simulink model "system_level_worst_case"  (R2025a)
settings: Solver=VariableStepAuto  StartTime=0.0  StopTime=350  RelTol=1e-3
libraries: simulink x5
settings Model: PacingRate=10  Creator=lynnyu  LastModifiedBy=lynnyu

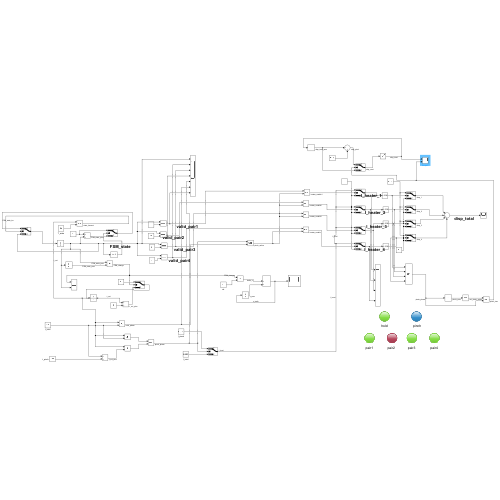
[thumbnail: Simulink's stored preview of the top-level diagram]
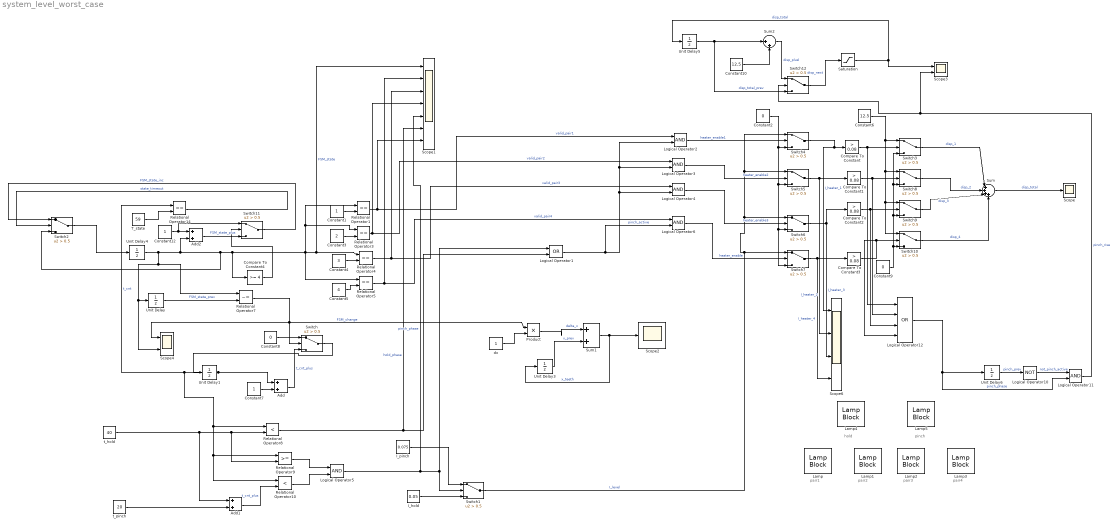
== system system_level_worst_case ==
  note: pair1
  note: pair2
  note: pair3
  note: pair4
  note: hold
  note: pinch
  Add : Sum
  Add1 : Sum
  Add2 : Sum
  Compare To Constant{,1..3} (4 alike) : simulink/Logic and Bit Operations/Compare To Constant  relop=>  const=0.08  OutDataTypeStr=boolean
  Compare To Constant4 : simulink/Logic and Bit Operations/Compare To Constant  relop=>=  const=4  OutDataTypeStr=boolean
  Constant1 : Constant
  Constant10 : Constant  Value=12.5
  Constant12 : Constant
  Constant2 : Constant  Value=0
  Constant3 : Constant  Value=2
  Constant4 : Constant  Value=3
  Constant5 : Constant  Value=4
  Constant6 : Constant  Value=12.5
  Constant7 : Constant
  Constant8 : Constant  Value=0
  Constant9 : Constant  Value=0
  I_hold : Constant  Value=0.05
  I_pinch : Constant  Value=0.075
  Lamp{,1..5} (6 alike) : LampBlock  LabelPosition=Hide  DefaultColor=[192.0, 192.0, 192.0]
  Logical Operator1 : Logic  Operator=OR  AllPortsSameDT=off  OutDataTypeStr=boolean
  Logical Operator10 : Logic  Operator=NOT  AllPortsSameDT=off  OutDataTypeStr=boolean
  Logical Operator{2..6,11} (6 alike) : Logic  AllPortsSameDT=off  OutDataTypeStr=boolean
  Logical Operator12 : Logic  Operator=OR  Inputs=4  AllPortsSameDT=off  OutDataTypeStr=boolean
  Product : Product
  Relational Operator{1,3..5,14} (5 alike) : RelationalOperator  Operator===  OutDataTypeStr=boolean  RndMeth=Simplest  InputSameDT=off
  Relational Operator10 : RelationalOperator  Operator=<  OutDataTypeStr=boolean  RndMeth=Simplest  InputSameDT=off
  Relational Operator7 : RelationalOperator  Operator=~=  OutDataTypeStr=boolean  RndMeth=Simplest  InputSameDT=off
  Relational Operator8 : RelationalOperator  Operator=<  OutDataTypeStr=boolean  RndMeth=Simplest  InputSameDT=off
  Relational Operator9 : RelationalOperator  OutDataTypeStr=boolean  RndMeth=Simplest  InputSameDT=off
  Saturation : Saturate  UpperLimit=50  LowerLimit=0
  Scope : Scope
      settings: ActiveDisplayYMinimum=-18.306271567614282  ActiveDisplayYMaximum=37.306576892811549
  Scope1 : Scope  NumInputPorts=7
      settings: ActiveDisplayYMinimum=-0.49999999999999989  ActiveDisplayYMaximum=4.5  DataLoggingVariableName=ScopeData2
  Scope2 : Scope
      settings: ActiveDisplayYMinimum=-19.976323121844477  ActiveDisplayYMaximum=15.328219620645053
  Scope3 : Scope  NumInputPorts=2
      settings: ActiveDisplayYMinimum=-6.2499999999999982  ActiveDisplayYMaximum=56.25  DataLoggingVariableName=ScopeData4
  Scope4 : Scope  NumInputPorts=2
      settings: ActiveDisplayYMinimum=-18.151033630505076  ActiveDisplayYMaximum=23.346420092188417  DataLoggingVariableName=ScopeData3
  Scope6 : Scope  NumInputPorts=4
      settings: ActiveDisplayYMinimum=-0.014999999999999996  ActiveDisplayYMaximum=0.135  DataLoggingVariableName=ScopeData6
  Sum : Sum  Inputs=|++++
  Sum1 : Sum  Inputs=|++
  Sum2 : Sum  Inputs=|++
  Switch{,1..12} (13 alike) : Switch  Criteria=u2 > Threshold  Threshold=0.5  SaturateOnIntegerOverflow=off  InputSameDT=off
  T_state : Constant  Value=59
  Unit Delay{,3,5..6} (4 alike) : UnitDelay  SampleTime=-1  HasFrameUpgradeWarning=on
  Unit Delay1 : UnitDelay  HasFrameUpgradeWarning=on
  Unit Delay4 : UnitDelay  InitialCondition=1  HasFrameUpgradeWarning=on
  dx : Constant
  t_hold : Constant  Value=40
  t_pinch : Constant  Value=20
  wires:
  Unit Delay4/1 -> Compare To Constant4/1, Scope1/1, Relational Operator4/1, Relational Operator5/1, Relational Operator3/1, Relational Operator1/1, Switch2/3, Add2/2, Scope4/2, Unit Delay/1, Relational Operator7/1  "FSM_state"
  Constant1/1 -> Relational Operator1/2
  Constant3/1 -> Relational Operator3/2
  Constant4/1 -> Relational Operator4/2
  Constant5/1 -> Relational Operator5/2
  Unit Delay1/1 -> Relational Operator9/1, Relational Operator10/1, Relational Operator8/1, Relational Operator14/1, Add/1  "t_cnt"
  Constant7/1 -> Add/2
  Add/1 -> Switch/3  "t_cnt_plus"
  Constant8/1 -> Switch/1
  Switch/1 -> Unit Delay1/1
  t_hold/1 -> Add1/1, Relational Operator8/2, Relational Operator9/2
  Relational Operator8/1 -> Scope1/6, Logical Operator1/2  "hold_phase"
  t_pinch/1 -> Add1/2
  Add1/1 -> Relational Operator10/2  "t_cnt_plus"
  Relational Operator9/1 -> Logical Operator5/1
  Relational Operator10/1 -> Logical Operator5/2
  I_pinch/1 -> Switch1/1
  I_hold/1 -> Switch1/3
  Switch1/1 -> Switch5/1, Switch4/1, Switch6/1, Switch7/1  "I_level"
  Relational Operator7/1 -> Switch/2, Product/1, Scope4/1  "FSM_change"
  dx/1 -> Product/2
  Product/1 -> Sum1/1  "delta_x"
  Unit Delay3/1 -> Sum1/2  "x_prev"
  Sum1/1 -> Unit Delay3/1, Scope2/1  "x_teeth"
  Unit Delay/1 -> Relational Operator7/2  "FSM_state_prev"
  Relational Operator14/1 -> Switch2/2  "state_timeout"
  Constant12/1 -> Switch11/1, Add2/1
  Add2/1 -> Switch11/3  "FSM_state_plus"
  Switch11/1 -> Switch2/1  "FSM_state_inc"
  Switch2/1 -> Unit Delay4/1
  T_state/1 -> Relational Operator14/2
  Relational Operator3/1 -> Logical Operator3/1, Scope1/4  "valid_pair2"
  Relational Operator4/1 -> Scope1/3, Logical Operator4/1  "valid_pair3"
  Relational Operator5/1 -> Scope1/2, Logical Operator6/1  "valid_pair4"
  Switch7/1 -> Compare To Constant3/1, Scope6/4  "I_heater_4"
  Logical Operator4/1 -> Switch6/2  "heater_enable3"
  Switch5/1 -> Scope6/2, Compare To Constant1/1  "I_heater_2"
  Constant2/1 -> Switch7/3, Switch6/3, Switch5/3, Switch4/3
  Logical Operator2/1 -> Switch4/2  "heater_enable1"
  Relational Operator1/1 -> Scope1/7, Logical Operator2/1  "valid_pair1"
  Logical Operator6/1 -> Switch7/2  "heater_enable"
  Logical Operator1/1 -> Logical Operator2/2, Logical Operator3/2, Logical Operator4/2, Logical Operator6/2  "pinch_active"
  Logical Operator3/1 -> Switch5/2  "heater_enable2"
  Switch4/1 -> Scope6/1, Compare To Constant/1  "I_heater_1"
  Switch6/1 -> Compare To Constant2/1, Scope6/3  "I_heater_3"
  Constant6/1 -> Switch10/1, Switch9/1, Switch8/1, Switch3/1
  Constant9/1 -> Switch10/3, Switch9/3, Switch8/3, Switch3/3
  Compare To Constant/1 -> Logical Operator12/1, Switch3/2
  Compare To Constant1/1 -> Logical Operator12/2, Switch8/2
  Compare To Constant2/1 -> Switch9/2, Logical Operator12/3
  Compare To Constant3/1 -> Switch10/2, Logical Operator12/4
  Switch3/1 -> Sum/1  "disp_1"
  Switch8/1 -> Sum/2  "disp_2"
  Switch10/1 -> Sum/4  "disp_4"
  Switch9/1 -> Sum/3  "disp_3"
  Sum/1 -> Scope/1  "disp_total"
  Compare To Constant4/1 -> Switch11/2
  Unit Delay5/1 -> Switch12/3, Sum2/1  "disp_total_prev"
  Constant10/1 -> Sum2/2
  Sum2/1 -> Switch12/1  "disp_plusl"
  Switch12/1 -> Saturation/1  "disp_next"
  Saturation/1 -> Unit Delay5/1, Scope3/1  "disp_total"
  Logical Operator5/1 -> Scope1/5, Switch1/2, Logical Operator1/1  "pinch_phase"
  Unit Delay6/1 -> Logical Operator10/1  "pinch_prev"
  Logical Operator12/1 -> Logical Operator11/2, Unit Delay6/1  "pinch_phase"
  Logical Operator10/1 -> Logical Operator11/1  "not_pinch_active"
  Logical Operator11/1 -> Scope3/2, Switch12/2  "pinch_rise"
